simulink library "Controllers"  (R2013a)
settings: Solver=ode45  StartTime=0.0  StopTime=10.0  RelTol=1e-3
settings Model: Creator=Felipe  LastModifiedBy=Felipe

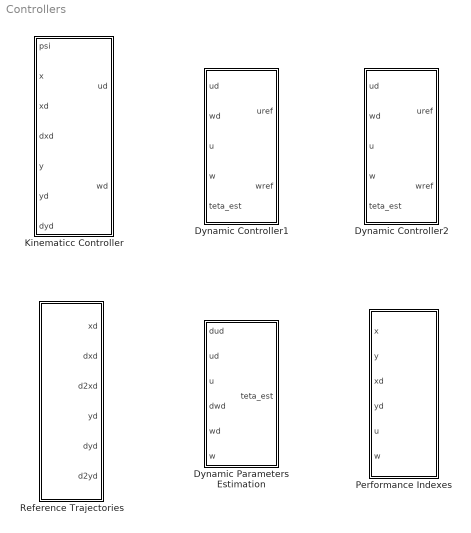
== system Controllers ==
  Dynamic Parameters Estimation : Subsystem  mask(Dynamic Parameters Estimation){ku=4, kw=4, lu=1, lw=1, inicia_adapt=50, theta=[0.30822 0.16922 -0.00058 0.80630 -0.00244 1.13994], gamma=[1.7 1.1 0.5 0.5 0.5 0.5], sig_mod=[0.0005 0.001 0.001 0.00006 0.001 0.000]}
      mask prompts: ku "Dynamic controller linear velocity gain: ku"; kw "Dynamic controller angular velocity gain: kw"; lu "Dynamic controller linear velocity saturation constant: lu"; lw "Dynamic controller angular velocity saturation constant: lw"; inicia_adapt "Time to begin parameter update: t[s]"; theta "Initial parameter estimates (1x6):"; gamma "Adaptation gains for parameter estimation (1x6):"; sig_mod "Sigma modification gains for parameter estimation (1x6):"
      mask help: This block implements a dynamic parameters estimatior to be used with the velocity-based dynamic compensation controller for differential-drive mobile robots.
      mask Help:
      | This block implements a dynamic parameters estimatior to be used with the velocity-based dynamic compensation controller for differential-drive mobile robots.
      | It receives the robot actual [u, w] and desired [ud, wd] values for linear and angular velocities, and the desired robot acceleration [dud, dwd]. Based on the velocity error, it adjusts the values of the estimated dynamic parameters [teta_est].
      | 
      | <b>Parameters:</b>
      | 
      | ku > 0 and kw > 0 are the dynamic controller gains.
      | lu > 0 and lw > 0 are the dynamic controller saturation constants.
      | t [s] (1x1): time to begin parameter update (before this time parameter estimates are kept constant)
      | gamma (1x6): adaptation gains for parameter estimation
      | Initial parameter estimates (1x6): Initial estimates for the dynamic parameters
      | 
      | <b>Inputs:</b>
      | 
      | dud (1x1): desired linear acceleration [m/s^2];
      | dwd (1x1): desired angular acceleration [rad/s^2];
      | ud (1x1): desired linear velocity [m/s] generated by the kinematic controller;
      | wd (1x1): desired angular velocity [rad/s] generated by the kinematic controller;
      | u (1x1): actual robot linear velocity [m/s];
      | w (1x1): actual robot angular velocity [rad/s];
      | 
      | 
      | <b>Outputs:</b>
      | 
      | teta_est (1x6): Estimated dynamic parameters for the mobile robot acoording to [1-3]:
      | [\theta_1 [s], \theta_2 [s], \theta_3 [sm/rad2], \theta_4, \theta_5 [s/m], \theta_6]
      | 
      | <b>Use:</b>
      | 
      | The inputs must recieve the reference signals for linear and angular velocities generated by a kinematic controller, and the actual robot linear and angular velocities.
      | The output [teta_est] is to be conected to a dynamic compensator controller.
      | 
      | <b>Notes:</b>
      | 
      | The following sets of parameters were obtained via identification for some differential-drive mobile robots:
      | 
      | [0.2604 0.2509 -0.000499 0.9965 0.00263 1.0768]; % Pioneer 3 with Sick LASER sensor
      | [0.5338 0.2168 -0.0134 0.9560 -0.0843 1.0590]; % Pioneer 3 without LASER sensor
      | [0.1992 0.13736 0.001954 0.9907 0.01554 0.9866]; % Pioneer 2 without onboard computer (no LASER sensor)
      | [0.3037 0.2768 -0.0004018 0.9835 0.003818 1.0725]; % Pioneer 2 with onboard computer (no LASER sensor)
      | [0.3759 0.0188 0.0128 1.0027 -0.0015 0.9808]; % Robotic wheelchair carring a 55kg person
      | [0.4263 0.0289 0.0058 0.9883 0.0134 0.9931]; % Robotic wheelchair carring a 125kg person
      | 
      | 
      | ------
      | For detailed information on the system, please refer to the following papers and thesis:
      | 
      | [1] MARTINS, F. N., Celeste, W. C., Carelli, R., Sarcinelli-Filho, M. and
      | Bastos-Filho, T. F. An Adaptive Dynamic Controller for Autonomous Mobile Robot
      | Trajectory Tracking. Control Engineering Practice, v. 16, p. 1354–1363, 2008.
      | doi: 10.1016/j.conengprac.2008.03.004
      | 
      | [2] MARTINS, F. N., Carelli, R., Sarcinelli-Filho, M. and Bastos-Filho, T. F.
      | Dynamic Modeling and Adaptive Dynamic Compensation for Unicycle-Like
      | Mobile Robots. 14th International Conference on Advanced Robotics -
      | ICAR 2009, Germany, June, 22-26, 2009.
      | 
      | [3] Thesis: "Modelagem e Compensacao da Dinamica de Robos Moveis e sua
      | Aplicacao em Controle de Formacao". Felipe Nascimento Martins. Tese de
      | Doutorado em Engenharia Eletrica - Automacao. UFES, 2009.
      | 
      | ---
      | Based on a prior work by Felipe Nascimento Martins and Wanderley Cardoso Celeste
      | UFES - Federal University of Espirito Santo, BRAZIL
      | 2006--2008
      | 
      | Author: Felipe Nascimento Martins
      | Federal Institute of Education, Science and Technology of Espirito Santo - IFES
      | NERA - Núcleo de Estudos em Robótica e Automação
      | http://nera.sr.ifes.edu.br
      | MAY/2013
      | Blog sobre robótica: www.nossosrobos.blogspot.com
  Dynamic Controller1 : Subsystem  mask(Dynamic Controller 1){ku=4, kw=4}
      mask prompts: ku "Linear velocity gain: ku"; kw "Angular velocity gain: kw"
      mask help: This block implements a velocity-based dynamic compensation controller for differential-drive mobile robots.
      mask Help:
      | This block implements a velocity-based dynamic compensation controller for differential-drive mobile robots.
      | It receives the references for linear and angular velocities [ud, wd] from the kinematic controller and generates another pair of linear and angular velocity commands [uref, wref] for the robot servos.
      | 
      | <b>Parameters:</b>
      | 
      | ku > 0 and kw > 0 are the controller gains.
      | 
      | <b>Inputs:</b>
      | 
      | ud (1x1): desired linear velocity [m/s] generated by the kinematic controller;
      | wd (1x1): desired angular velocity [rad/s] generated by the kinematic controller;
      | u (1x1): actual robot linear velocity [m/s];
      | w (1x1): actual robot angular velocity [rad/s];
      | teta_est (1x6): Estimated dynamic parameters for an specific mobile robot acoording to [1-3]:
      | [\theta_1 [s], \theta_2 [s], \theta_3 [sm/rad2], \theta_4, \theta_5 [s/m], \theta_6]
      | 
      | 
      | <b>Outputs:</b>
      | 
      | uref (1x1): reference for linear velocity [m/s]
      | wref (1x1): reference for angular velocity [rad/s]
      | 
      | <b>Use:</b>
      | 
      | The inputs must recieve the reference signals for linear and angular velocities generated by a kinematic controller, and the actual robot linear and angular velocities.
      | In order to perform correct dynamic compensation, the (1x6) vector of estimated dynamic parameters must be provided. This vector can be constant or can vary according to an adaptation rule.
      | 
      | The outputs [vref, wref] are to be conected to the robot.
      | 
      | 
      | <b>Notes:</b>
      | 
      | The following sets of parameters were obtained via identification for some differential-drive mobile robots:
      | 
      | [0.2604 0.2509 -0.000499 0.9965 0.00263 1.0768]; % Pioneer 3 with Sick LASER sensor
      | [0.5338 0.2168 -0.0134 0.9560 -0.0843 1.0590]; % Pioneer 3 without LASER sensor
      | [0.1992 0.13736 0.001954 0.9907 0.01554 0.9866]; % Pioneer 2 without onboard computer (no LASER sensor)
      | [0.3037 0.2768 -0.0004018 0.9835 0.003818 1.0725]; % Pioneer 2 with onboard computer (no LASER sensor)
      | [0.3759 0.0188 0.0128 1.0027 -0.0015 0.9808]; % Robotic wheelchair carring a 55kg person
      | [0.4263 0.0289 0.0058 0.9883 0.0134 0.9931]; % Robotic wheelchair carring a 125kg person
      | 
      | 
      | ------
      | For detailed information on the system, please refer to the following papers and thesis:
      | 
      | [1] MARTINS, F. N., Celeste, W. C., Carelli, R., Sarcinelli-Filho, M. and
      | Bastos-Filho, T. F. An Adaptive Dynamic Controller for Autonomous Mobile Robot
      | Trajectory Tracking. Control Engineering Practice, v. 16, p. 1354–1363, 2008.
      | doi: 10.1016/j.conengprac.2008.03.004
      | 
      | [2] MARTINS, F. N., Carelli, R., Sarcinelli-Filho, M. and Bastos-Filho, T. F.
      | Dynamic Modeling and Adaptive Dynamic Compensation for Unicycle-Like
      | Mobile Robots. 14th International Conference on Advanced Robotics -
      | ICAR 2009, Germany, June, 22-26, 2009.
      | 
      | [3] Thesis: "Modelagem e Compensacao da Dinamica de Robos Moveis e sua
      | Aplicacao em Controle de Formacao". Felipe Nascimento Martins. Tese de
      | Doutorado em Engenharia Eletrica - Automacao. UFES, 2009.
      | 
      | ---
      | Based on a prior work by Felipe Nascimento Martins and Wanderley Cardoso Celeste
      | UFES - Federal University of Espirito Santo, BRAZIL
      | 2006--2008
      | 
      | Author: Felipe Nascimento Martins
      | Federal Institute of Education, Science and Technology of Espirito Santo - IFES
      | NERA - Núcleo de Estudos em Robótica e Automação
      | http://nera.sr.ifes.edu.br
      | MAY/2013
      | Blog sobre robótica: www.nossosrobos.blogspot.com
  Dynamic Controller2 : Subsystem  mask(Dynamic Controller 2){ku=4, kw=4, lu=1, lw=1}
      mask prompts: ku "Linear velocity gain: ku"; kw "Angular velocity gain: kw"; lu "Linear velocity saturation constant: lu"; lw "Angular velocity saturation constant: lw"
      mask help: This block implements a velocity-based dynamic compensation controller for differential-drive mobile robots.
      mask Help:
      | This block implements a velocity-based dynamic compensation controller for differential-drive mobile robots.
      | It receives the references for linear and angular velocities [ud, wd] from the kinematic controller and generates another pair of linear and angular velocity commands [uref, wref] for the robot servos.
      | 
      | <b>Parameters:</b>
      | 
      | ku > 0 and kw > 0 are the controller gains.
      | lu > 0 and lw > 0 are saturation constants.
      | 
      | <b>Inputs:</b>
      | 
      | ud (1x1): desired linear velocity [m/s] generated by the kinematic controller;
      | wd (1x1): desired angular velocity [rad/s] generated by the kinematic controller;
      | u (1x1): actual robot linear velocity [m/s];
      | w (1x1): actual robot angular velocity [rad/s];
      | teta_est (1x6): Estimated dynamic parameters for an specific mobile robot acoording to [1-3]:
      | [\theta_1 [s], \theta_2 [s], \theta_3 [sm/rad2], \theta_4, \theta_5 [s/m], \theta_6]
      | 
      | 
      | <b>Outputs:</b>
      | 
      | uref (1x1): reference for linear velocity [m/s]
      | wref (1x1): reference for angular velocity [rad/s]
      | 
      | <b>Use:</b>
      | 
      | The inputs must recieve the reference signals for linear and angular velocities generated by a kinematic controller, and the actual robot linear and angular velocities.
      | In order to perform correct dynamic compensation, the (1x6) vector of estimated dynamic parameters must be provided. This vector can be constant or can vary according to an adaptation rule.
      | 
      | The outputs [vref, wref] are to be conected to the robot.
      | 
      | 
      | <b>Notes:</b>
      | 
      | The following sets of parameters were obtained via identification for some differential-drive mobile robots:
      | 
      | [0.2604 0.2509 -0.000499 0.9965 0.00263 1.0768]; % Pioneer 3 with Sick LASER sensor
      | [0.5338 0.2168 -0.0134 0.9560 -0.0843 1.0590]; % Pioneer 3 without LASER sensor
      | [0.1992 0.13736 0.001954 0.9907 0.01554 0.9866]; % Pioneer 2 without onboard computer (no LASER sensor)
      | [0.3037 0.2768 -0.0004018 0.9835 0.003818 1.0725]; % Pioneer 2 with onboard computer (no LASER sensor)
      | [0.3759 0.0188 0.0128 1.0027 -0.0015 0.9808]; % Robotic wheelchair carring a 55kg person
      | [0.4263 0.0289 0.0058 0.9883 0.0134 0.9931]; % Robotic wheelchair carring a 125kg person
      | 
      | 
      | ------
      | For detailed information on the system, please refer to the following papers and thesis:
      | 
      | [1] MARTINS, F. N., Celeste, W. C., Carelli, R., Sarcinelli-Filho, M. and
      | Bastos-Filho, T. F. An Adaptive Dynamic Controller for Autonomous Mobile Robot
      | Trajectory Tracking. Control Engineering Practice, v. 16, p. 1354–1363, 2008.
      | doi: 10.1016/j.conengprac.2008.03.004
      | 
      | [2] MARTINS, F. N., Carelli, R., Sarcinelli-Filho, M. and Bastos-Filho, T. F.
      | Dynamic Modeling and Adaptive Dynamic Compensation for Unicycle-Like
      | Mobile Robots. 14th International Conference on Advanced Robotics -
      | ICAR 2009, Germany, June, 22-26, 2009.
      | 
      | [3] Thesis: "Modelagem e Compensacao da Dinamica de Robos Moveis e sua
      | Aplicacao em Controle de Formacao". Felipe Nascimento Martins. Tese de
      | Doutorado em Engenharia Eletrica - Automacao. UFES, 2009.
      | 
      | ---
      | Based on a prior work by Felipe Nascimento Martins and Wanderley Cardoso Celeste
      | UFES - Federal University of Espirito Santo, BRAZIL
      | 2006--2008
      | 
      | Author: Felipe Nascimento Martins
      | Federal Institute of Education, Science and Technology of Espirito Santo - IFES
      | NERA - Núcleo de Estudos em Robótica e Automação
      | http://nera.sr.ifes.edu.br
      | MAY/2013
      | Blog sobre robótica: www.nossosrobos.blogspot.com
  Kinematicc Controller : Subsystem  mask(Kinematic Controller){kx=4, ky=4, lx=4, ly=4, a=0.2}
      mask prompts: kx "Controller gain: kx"; ky "Controller gain: ky"; lx "Saturation constant: lx"; ly "Saturation constant: ly"; a "Distance from the the point of interest to the center of the line that connects the traction wheels [m]"
      mask help: This block implements a controller for differential-drive mobile robots to follow a desired trajectory or to go to a goal point.
      mask Help:
      | This block implements a controller for differential-drive mobile robots to follow a desired trajectory or to go to a goal point.
      | 
      | The trajectory tracking controller is based on the inverse kinematics of the differential-drive robot, whereas only the position [x, y] of the point of interest is considered.
      | It generates references for linear and angular velocities [ud, wd] based on the robot's actual pose [x, y, psi] deseired position [xd, yd] and desired speed [dxd, dyd].
      | 
      | The constant "a" represents the distance of the point of interest [x, y] to the center of the line that connects the traction wheels.
      | 
      | <b>Parameters:</b>
      | 
      | kx > 0 and ky > 0: controller gains;
      | lx > 0 and ly > 0: saturation constants.
      | 
      | 
      | <b>Inputs:</b>
      | 
      | psi: actual robot orientation [rad] (psi=0 means the robot orientation is the same as the x axis);
      | x: actual robot position [m] in x axis;
      | xd: desired robot position [m] in x axis;
      | dxd: desired robot speed [m/s] in x axis;
      | y: actual robot position [m] in y axis;
      | yd: desired robot position [m] in y axis;
      | dyd: desired robot speed [m/s] in y axis;
      | 
      | <b>Outputs:</b>
      | 
      | ud: reference for linear velocity [m/s]
      | wd: reference for angular velocity [rad/s]
      | 
      | 
      | <b>Notes:</b>
      | 
      | If the deseired position [xd, yd] is constant and the desired speed [dxd, dyd] is zero, the controller works as a position controller: it drives the robot to a goal position [xd, yd].
      | 
      | ------
      | For detailed information on the system, please refer to the following papers and thesis:
      | 
      | [1] MARTINS, F. N., Celeste, W. C., Carelli, R., Sarcinelli-Filho, M. and
      | Bastos-Filho, T. F. An Adaptive Dynamic Controller for Autonomous Mobile Robot
      | Trajectory Tracking. Control Engineering Practice, v. 16, p. 1354–1363, 2008.
      | doi: 10.1016/j.conengprac.2008.03.004
      | 
      | [2] MARTINS, F. N., Carelli, R., Sarcinelli-Filho, M. and Bastos-Filho, T. F.
      | Dynamic Modeling and Adaptive Dynamic Compensation for Unicycle-Like
      | Mobile Robots. 14th International Conference on Advanced Robotics -
      | ICAR 2009, Germany, June, 22-26, 2009.
      | 
      | [3] Thesis: "Modelagem e Compensacao da Dinamica de Robos Moveis e sua
      | Aplicacao em Controle de Formacao". Felipe Nascimento Martins. Tese de
      | Doutorado em Engenharia Eletrica - Automacao. UFES, 2009.
      | 
      | ---
      | Based on a prior work by Felipe Nascimento Martins and Wanderley Cardoso Celeste
      | UFES - Federal University of Espirito Santo, BRAZIL
      | 2006--2008
      | 
      | Author: Felipe Nascimento Martins
      | Federal Institute of Education, Science and Technology of Espirito Santo - IFES
      | NERA - Núcleo de Estudos em Robótica e Automação
      | http://nera.sr.ifes.edu.br
      | MAY/2013
      | Blog sobre robótica: www.nossosrobos.blogspot.com
  Performance Indexes : Subsystem  mask(Performance Indexes){}
      mask help:
      | Calcultes the following performance indexes: IAE, ITAE, ISE, ITSE. Also calculates an Energy-based index.
      | Results are transfered to workspace variables: iae, itae, ise, itse, energy.
      mask Help:
      | Calcultes the following performance indexes: IAE, ITAE, ISE, ITSE. Also calculates an Energy-based index.
      | This block is intended to be used with mobile robot model and controllers in order to provide information to compare the performance of different controllers and gain sets.
      | 
      | Inputs:
      | x: actual robot position in x
      | y: actual robot position in y
      | xd: desired robot position in x
      | yd: desired robot position in y
      | u: actual robot linear velocity
      | w: actual robot angular velocity
      | 
      | Outputs:
      | Results are transfered to workspace variables: iae, itae, ise, itse, energy.
  Reference Trajectories : Subsystem  mask(Reference Trajectories){trajectory_type=2, wf=0.10, raio_ref_1=1, delta_raio=-0.1, t_delta_raio=60, xd=[2, 3]}
      mask prompts: trajectory_type "Trajectory type: 1=Circle, 2=Eight, 3=Line, 4=Fixed Point"; wf "Angular speed for circle and eight [rad/s]"; raio_ref_1 "Radius for circle and eight (each side) [m]"; delta_raio "Radius variation (circle only)"; t_delta_raio "Time between radius variation (circle only) [s]"; xd "Goal position (for fixed point only) (1x2)"
      mask help: Generates reference values of position, velocity and acceleration.
      mask Help:
      | Generates reference values of position, velocity and acceleration.
      | This block is intended to be used with mobile robot trajectory tracking kinematic controller.
      | 
      | Available references:
      | - Circular trajectory with 2 different radius;
      | - Eight-shape trajectory;
      | - Linear trajectory;
      | - Fixed point.
      | 
      | 
      | <b> Parameters:</b>
      | 
      | Trajectory type: 1=Circle, 2=Eight, 3=Line, 4=Fixed Point
      | Angular speed for circle and eight (1x1) [rad/s]
      | Radius for circle and eight (each side) (1x1)[m]
      | Radius variation (circle only) delta_raio (1x1) [m]
      | Time between radius variation (circle only) (1x1) [s]
      | 
      | <b> Outputs: </b>
      | 
      | xd: desired robot position [m] in x axis;
      | dxd: desired robot speed [m/s] in x axis;
      | d2xd: desired robot acceleration [m/s^2] in x axis;
      | yd: desired robot position [m] in y axis;
      | dyd: desired robot speed [m/s] in y axis;
      | d2yd: desired robot acceleration [m/s^2] in y axis;

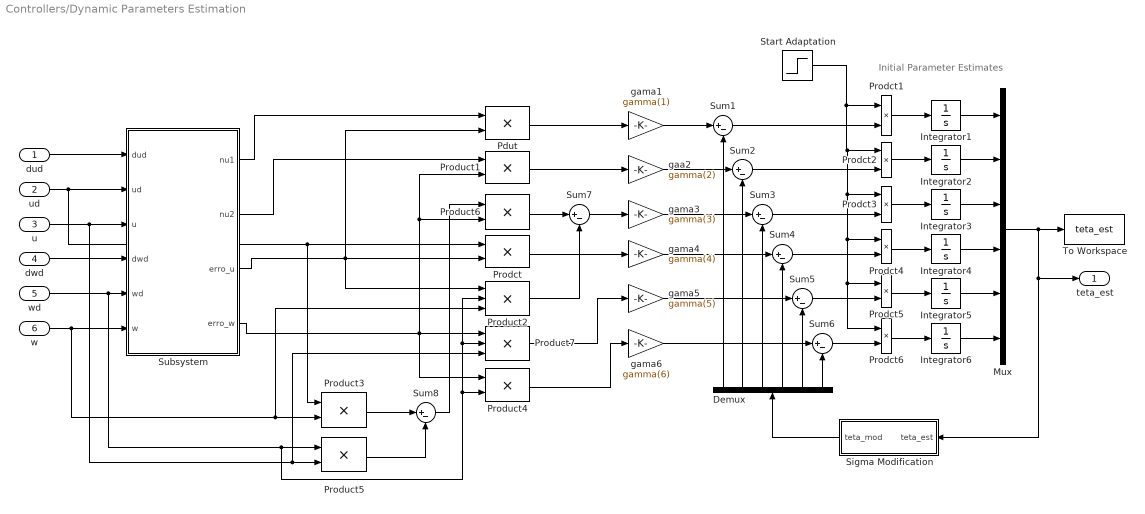
== system Controllers/Dynamic Parameters Estimation ==
  note: Initial Parameter
      | Estimates
  dud : Inport
  ud : Inport  Port=2
  u : Inport  Port=3
  dwd : Inport  Port=4
  wd : Inport  Port=5
  w : Inport  Port=6
  Demux : Demux  Outputs=6
  Integrator1 : Integrator  InitialCondition=theta(1)
  Integrator2 : Integrator  InitialCondition=theta(2)
  Integrator3 : Integrator  InitialCondition=theta(3)
  Integrator4 : Integrator  InitialCondition=theta(4)
  Integrator5 : Integrator  InitialCondition=theta(5)
  Integrator6 : Integrator  InitialCondition=theta(6)
  Mux : Mux  Inputs=6
  Pdut : Product  SaturateOnIntegerOverflow=on  OutDataTypeStr=Inherit: Same as first input
  Prodct{,1..6} (7 alike) : Product  SaturateOnIntegerOverflow=on  OutDataTypeStr=Inherit: Same as first input
  Product{1,3..6} (5 alike) : Product  SaturateOnIntegerOverflow=on  OutDataTypeStr=Inherit: Same as first input
  Product2 : Product  Inputs=3  SaturateOnIntegerOverflow=on  OutDataTypeStr=Inherit: Same as first input
  Product7 : Product  Inputs=3  SaturateOnIntegerOverflow=on  OutDataTypeStr=Inherit: Same as first input
  Sigma Modification : Subsystem
  Start Adaptation : Step  Time=inicia_adapt  SampleTime=0
  Subsystem : Subsystem
  Sum{1..8} (8 alike) : Sum  Inputs=|+-  SaturateOnIntegerOverflow=on
  To Workspace : ToWorkspace  VariableName=teta_est  SampleTime=-1
  gaa2 : Gain  Gain=gamma(2)  SaturateOnIntegerOverflow=on  OutDataTypeStr=Inherit: Same as input  ParamDataTypeStr=Inherit: Same as input
  gama1 : Gain  Gain=gamma(1)  SaturateOnIntegerOverflow=on  OutDataTypeStr=Inherit: Same as input  ParamDataTypeStr=Inherit: Same as input
  gama3 : Gain  Gain=gamma(3)  SaturateOnIntegerOverflow=on  OutDataTypeStr=Inherit: Same as input  ParamDataTypeStr=Inherit: Same as input
  gama4 : Gain  Gain=gamma(4)  SaturateOnIntegerOverflow=on  OutDataTypeStr=Inherit: Same as input  ParamDataTypeStr=Inherit: Same as input
  gama5 : Gain  Gain=gamma(5)  SaturateOnIntegerOverflow=on  OutDataTypeStr=Inherit: Same as input  ParamDataTypeStr=Inherit: Same as input
  gama6 : Gain  Gain=gamma(6)  SaturateOnIntegerOverflow=on  OutDataTypeStr=Inherit: Same as input  ParamDataTypeStr=Inherit: Same as input
  teta_est : Outport
  wires:
  dud/1 -> Subsystem/1(dud)
  dwd/1 -> Subsystem/4(dwd)
  Subsystem/1(nu1) -> Pdut/1
  Subsystem/2(nu2) -> Product1/1
  Pdut/1 -> gama1/1
  Product1/1 -> gaa2/1
  Prodct/1 -> gama4/1
  Product4/1 -> gama6/1
  Integrator1/1 -> Mux/1
  Integrator2/1 -> Mux/2
  Integrator3/1 -> Mux/3
  Integrator4/1 -> Mux/4
  Integrator5/1 -> Mux/5
  Integrator6/1 -> Mux/6
  Mux/1 -> To Workspace/1, teta_est/1, Sigma Modification/1(teta_est)
  Prodct1/1 -> Integrator1/1
  Prodct2/1 -> Integrator2/1
  Prodct3/1 -> Integrator3/1
  Prodct4/1 -> Integrator4/1
  Prodct5/1 -> Integrator5/1
  Prodct6/1 -> Integrator6/1
  Sigma Modification/1(teta_mod) -> Demux/1
  Sum1/1 -> Prodct1/2
  gama1/1 -> Sum1/1
  Demux/1 -> Sum1/2
  gaa2/1 -> Sum2/1
  Sum2/1 -> Prodct2/2
  Demux/2 -> Sum2/2
  Sum3/1 -> Prodct3/2
  gama3/1 -> Sum3/1
  Demux/3 -> Sum3/2
  gama4/1 -> Sum4/1
  Sum4/1 -> Prodct4/2
  Demux/4 -> Sum4/2
  Sum5/1 -> Prodct5/2
  gama5/1 -> Sum5/1
  Demux/5 -> Sum5/2
  gama6/1 -> Sum6/1
  Demux/6 -> Sum6/2
  Sum6/1 -> Prodct6/2
  Sum7/1 -> gama3/1
  Product2/1 -> Sum7/2
  Product3/1 -> Sum8/1
  Product5/1 -> Sum8/2
  Sum8/1 -> Product6/1
  Product6/1 -> Sum7/1
  Product7/1 -> gama5/1
  Start Adaptation/1 -> Prodct4/1, Prodct5/1, Prodct6/1, Prodct3/1, Prodct2/1, Prodct1/1
  ud/1 -> Subsystem/2(ud), Product3/1, Prodct/1
  u/1 -> Product7/3, Product5/2, Subsystem/3(u)
  wd/1 -> Product4/2, Product7/2, Product2/2, Product5/1, Subsystem/5(wd)
  w/1 -> Product2/3, Product3/2, Subsystem/6(w)
  Subsystem/3(erro_u) -> Product2/1, Pdut/2, Prodct/2
  Subsystem/4(erro_w) -> Product1/2, Product6/2, Product4/1, Product7/1

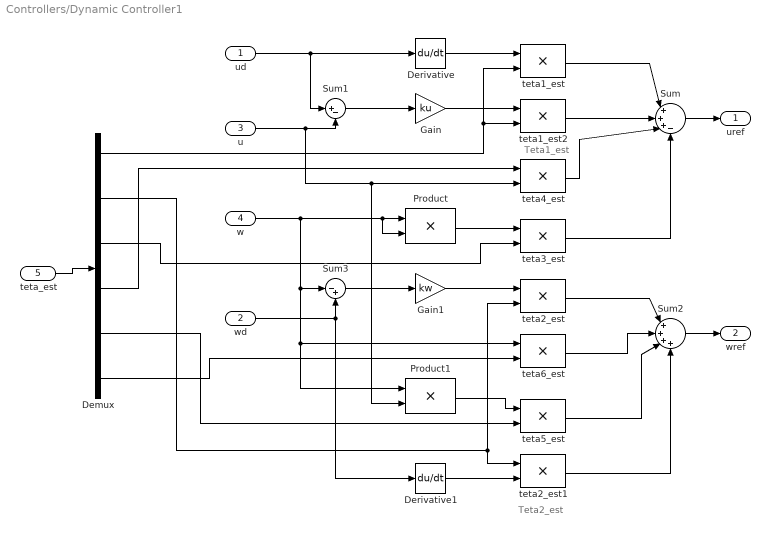
== system Controllers/Dynamic Controller1 ==
  note: Teta2_est
  note: Teta1_est
  ud : Inport
  wd : Inport  Port=2
  u : Inport  Port=3
  w : Inport  Port=4
  teta_est : Inport  Port=5
  Demux : Demux  Outputs=6
  Derivative : Derivative
  Derivative1 : Derivative
  Gain : Gain  Gain=ku  SaturateOnIntegerOverflow=on  OutDataTypeStr=Inherit: Same as input  ParamDataTypeStr=Inherit: Same as input
  Gain1 : Gain  Gain=kw  SaturateOnIntegerOverflow=on  OutDataTypeStr=Inherit: Same as input  ParamDataTypeStr=Inherit: Same as input
  Product : Product  SaturateOnIntegerOverflow=on  OutDataTypeStr=Inherit: Same as first input
  Product1 : Product  SaturateOnIntegerOverflow=on  OutDataTypeStr=Inherit: Same as first input
  Sum : Sum  Inputs=|+++-  SaturateOnIntegerOverflow=on
  Sum1 : Sum  Inputs=|+-  SaturateOnIntegerOverflow=on
  Sum2 : Sum  Inputs=|++++  SaturateOnIntegerOverflow=on
  Sum3 : Sum  Inputs=|-+  SaturateOnIntegerOverflow=on
  teta1_est : Product  SaturateOnIntegerOverflow=on  OutDataTypeStr=Inherit: Same as first input
  teta1_est2 : Product  SaturateOnIntegerOverflow=on  OutDataTypeStr=Inherit: Same as first input
  teta2_est : Product  SaturateOnIntegerOverflow=on  OutDataTypeStr=Inherit: Same as first input
  teta2_est1 : Product  SaturateOnIntegerOverflow=on  OutDataTypeStr=Inherit: Same as first input
  teta3_est : Product  SaturateOnIntegerOverflow=on  OutDataTypeStr=Inherit: Same as first input
  teta4_est : Product  SaturateOnIntegerOverflow=on  OutDataTypeStr=Inherit: Same as first input
  teta5_est : Product  SaturateOnIntegerOverflow=on  OutDataTypeStr=Inherit: Same as first input
  teta6_est : Product  SaturateOnIntegerOverflow=on  OutDataTypeStr=Inherit: Same as first input
  uref : Outport
  wref : Outport  Port=2
  wires:
  Sum/1 -> uref/1
  Sum2/1 -> wref/1
  Sum1/1 -> Gain/1
  teta1_est/1 -> Sum/1
  Product/1 -> teta3_est/1
  teta3_est/1 -> Sum/4
  Sum3/1 -> Gain1/1
  teta6_est/1 -> Sum2/2
  Product1/1 -> teta5_est/1
  teta1_est2/1 -> Sum/2
  teta_est/1 -> Demux/1
  teta4_est/1 -> Sum/3
  Demux/3 -> teta3_est/2
  teta2_est/1 -> Sum2/1
  Demux/6 -> teta6_est/2
  teta5_est/1 -> Sum2/3
  Demux/5 -> teta5_est/2
  teta2_est1/1 -> Sum2/4
  Derivative/1 -> teta1_est/1
  Derivative1/1 -> teta2_est1/2
  Gain/1 -> teta1_est2/1
  Gain1/1 -> teta2_est/1
  Demux/1 -> teta1_est/2, teta1_est2/2
  ud/1 -> Sum1/1, Derivative/1
  u/1 -> Sum1/2, teta4_est/2, Product1/2
  w/1 -> teta6_est/1, Product1/1, Sum3/1, Product/2, Product/1
  wd/1 -> Derivative1/1, Sum3/2
  Demux/2 -> teta2_est/2, teta2_est1/1
  Demux/4 -> teta4_est/1

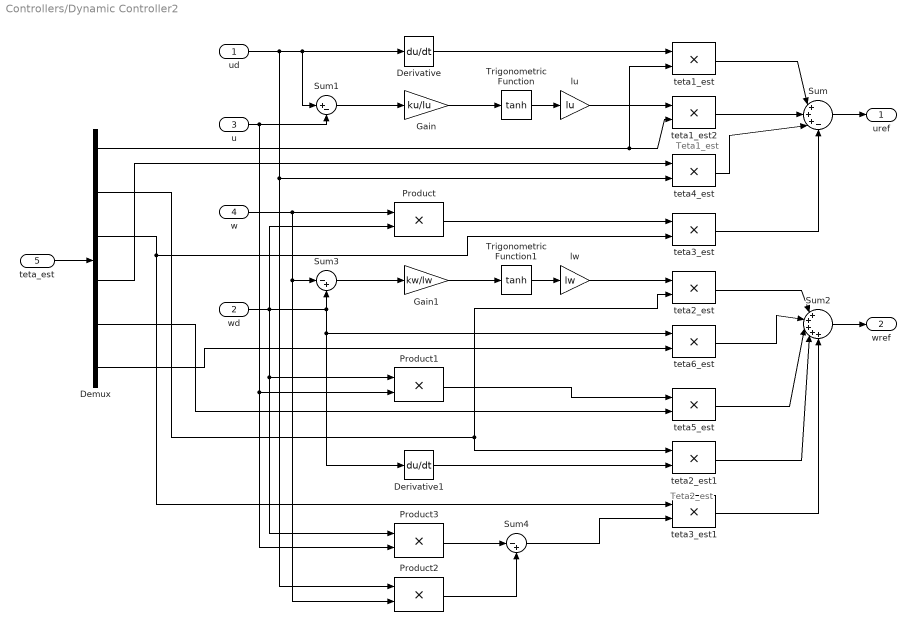
== system Controllers/Dynamic Controller2 ==
  note: Teta2_est
  note: Teta1_est
  ud : Inport
  wd : Inport  Port=2
  u : Inport  Port=3
  w : Inport  Port=4
  teta_est : Inport  Port=5
  Demux : Demux  Outputs=6
  Derivative : Derivative
  Derivative1 : Derivative
  Gain : Gain  Gain=ku/lu  SaturateOnIntegerOverflow=on  OutDataTypeStr=Inherit: Same as input  ParamDataTypeStr=Inherit: Same as input
  Gain1 : Gain  Gain=kw/lw  SaturateOnIntegerOverflow=on  OutDataTypeStr=Inherit: Same as input  ParamDataTypeStr=Inherit: Same as input
  Product{,1..3} (4 alike) : Product  SaturateOnIntegerOverflow=on  OutDataTypeStr=Inherit: Same as first input
  Sum : Sum  Inputs=|+++-  SaturateOnIntegerOverflow=on
  Sum1 : Sum  Inputs=|+-  SaturateOnIntegerOverflow=on
  Sum2 : Sum  Inputs=|+++++  SaturateOnIntegerOverflow=on
  Sum3 : Sum  Inputs=|-+  SaturateOnIntegerOverflow=on
  Sum4 : Sum  Inputs=|-+  SaturateOnIntegerOverflow=on
  Trigonometric Function : Trigonometry  Operator=tanh
  Trigonometric Function1 : Trigonometry  Operator=tanh
  lu : Gain  Gain=lu  SaturateOnIntegerOverflow=on  OutDataTypeStr=Inherit: Same as input  ParamDataTypeStr=Inherit: Same as input
  lw : Gain  Gain=lw  SaturateOnIntegerOverflow=on  OutDataTypeStr=Inherit: Same as input  ParamDataTypeStr=Inherit: Same as input
  teta1_est : Product  SaturateOnIntegerOverflow=on  OutDataTypeStr=Inherit: Same as first input
  teta1_est2 : Product  SaturateOnIntegerOverflow=on  OutDataTypeStr=Inherit: Same as first input
  teta2_est : Product  SaturateOnIntegerOverflow=on  OutDataTypeStr=Inherit: Same as first input
  teta2_est1 : Product  SaturateOnIntegerOverflow=on  OutDataTypeStr=Inherit: Same as first input
  teta3_est : Product  SaturateOnIntegerOverflow=on  OutDataTypeStr=Inherit: Same as first input
  teta3_est1 : Product  SaturateOnIntegerOverflow=on  OutDataTypeStr=Inherit: Same as first input
  teta4_est : Product  SaturateOnIntegerOverflow=on  OutDataTypeStr=Inherit: Same as first input
  teta5_est : Product  SaturateOnIntegerOverflow=on  OutDataTypeStr=Inherit: Same as first input
  teta6_est : Product  SaturateOnIntegerOverflow=on  OutDataTypeStr=Inherit: Same as first input
  uref : Outport
  wref : Outport  Port=2
  wires:
  Sum/1 -> uref/1
  Sum2/1 -> wref/1
  Sum1/1 -> Gain/1
  teta1_est/1 -> Sum/1
  Product/1 -> teta3_est/1
  teta3_est/1 -> Sum/4
  Sum3/1 -> Gain1/1
  teta6_est/1 -> Sum2/2
  Product1/1 -> teta5_est/1
  teta1_est2/1 -> Sum/2
  teta_est/1 -> Demux/1
  teta4_est/1 -> Sum/3
  Demux/3 -> teta3_est1/1, teta3_est/2
  teta2_est/1 -> Sum2/1
  Demux/6 -> teta6_est/2
  teta5_est/1 -> Sum2/3
  Demux/5 -> teta5_est/2
  teta2_est1/1 -> Sum2/4
  Derivative/1 -> teta1_est/1
  Derivative1/1 -> teta2_est1/2
  Demux/1 -> teta1_est/2, teta1_est2/2
  ud/1 -> Product2/1, teta4_est/2, Sum1/1, Derivative/1
  u/1 -> Sum1/2, Product3/2, Product1/2
  w/1 -> Product2/2, Sum3/1, Product/1
  wd/1 -> Product3/1, Product1/1, Product/2, teta6_est/1, Derivative1/1, Sum3/2
  Demux/2 -> teta2_est/2, teta2_est1/1
  Demux/4 -> teta4_est/1
  Trigonometric Function/1 -> lu/1
  lu/1 -> teta1_est2/1
  Gain/1 -> Trigonometric Function/1
  Trigonometric Function1/1 -> lw/1
  lw/1 -> teta2_est/1
  Gain1/1 -> Trigonometric Function1/1
  teta3_est1/1 -> Sum2/5
  Sum4/1 -> teta3_est1/2
  Product3/1 -> Sum4/1
  Product2/1 -> Sum4/2

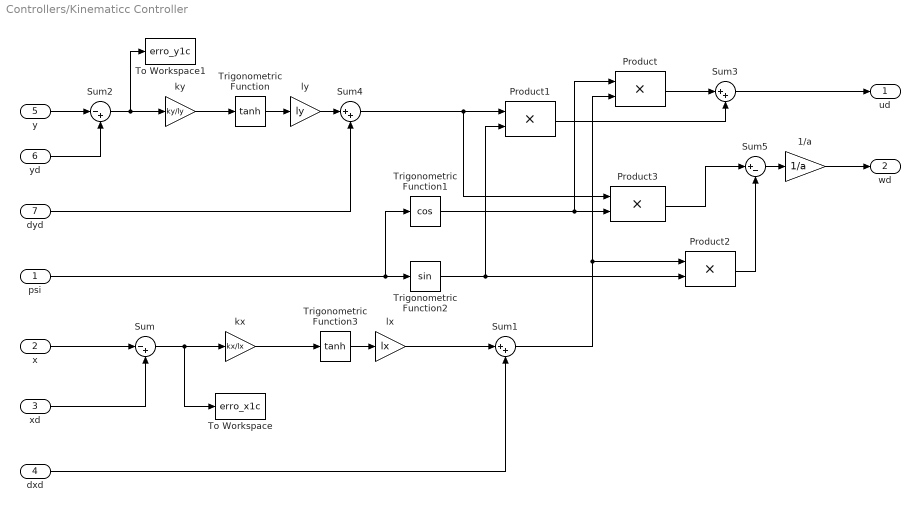
== system Controllers/Kinematicc Controller ==
  psi : Inport
  x : Inport  Port=2
  xd : Inport  Port=3
  dxd : Inport  Port=4
  y : Inport  Port=5
  yd : Inport  Port=6
  dyd : Inport  Port=7
  1/a : Gain  Gain=1/a  SaturateOnIntegerOverflow=on  OutDataTypeStr=Inherit: Same as input  ParamDataTypeStr=Inherit: Same as input
  Product{,1..3} (4 alike) : Product  SaturateOnIntegerOverflow=on  OutDataTypeStr=Inherit: Same as first input
  Sum : Sum  Inputs=|-+  SaturateOnIntegerOverflow=on
  Sum1 : Sum  Inputs=|++  SaturateOnIntegerOverflow=on
  Sum2 : Sum  Inputs=|-+  SaturateOnIntegerOverflow=on
  Sum3 : Sum  Inputs=|++  SaturateOnIntegerOverflow=on
  Sum4 : Sum  Inputs=|++  SaturateOnIntegerOverflow=on
  Sum5 : Sum  Inputs=|+-  SaturateOnIntegerOverflow=on
  To Workspace : ToWorkspace  VariableName=erro_x1c  SampleTime=-1
  To Workspace1 : ToWorkspace  VariableName=erro_y1c  SampleTime=-1
  Trigonometric Function : Trigonometry  Operator=tanh
  Trigonometric Function1 : Trigonometry  Operator=cos
  Trigonometric Function2 : Trigonometry
  Trigonometric Function3 : Trigonometry  Operator=tanh
  kx : Gain  Gain=kx/lx  SaturateOnIntegerOverflow=on  OutDataTypeStr=Inherit: Same as input  ParamDataTypeStr=Inherit: Same as input
  ky : Gain  Gain=ky/ly  SaturateOnIntegerOverflow=on  OutDataTypeStr=Inherit: Same as input  ParamDataTypeStr=Inherit: Same as input
  lx : Gain  Gain=lx  SaturateOnIntegerOverflow=on  OutDataTypeStr=Inherit: Same as input  ParamDataTypeStr=Inherit: Same as input
  ly : Gain  Gain=ly  SaturateOnIntegerOverflow=on  OutDataTypeStr=Inherit: Same as input  ParamDataTypeStr=Inherit: Same as input
  ud : Outport
  wd : Outport  Port=2
  wires:
  Sum5/1 -> 1/a/1
  Product2/1 -> Sum5/2
  Product3/1 -> Sum5/1
  Product1/1 -> Sum3/2
  Product/1 -> Sum3/1
  Sum2/1 -> To Workspace1/1, ky/1
  Sum1/1 -> Product/2, Product2/1
  psi/1 -> Trigonometric Function1/1, Trigonometric Function2/1
  x/1 -> Sum/1
  xd/1 -> Sum/2
  yd/1 -> Sum2/2
  Trigonometric Function3/1 -> lx/1
  lx/1 -> Sum1/1
  Trigonometric Function/1 -> ly/1
  ly/1 -> Sum4/1
  dyd/1 -> Sum4/2
  dxd/1 -> Sum1/2
  Sum3/1 -> ud/1
  1/a/1 -> wd/1
  Trigonometric Function2/1 -> Product1/2, Product2/2
  Sum4/1 -> Product3/1, Product1/1
  y/1 -> Sum2/1
  Sum/1 -> To Workspace/1, kx/1
  Trigonometric Function1/1 -> Product/1, Product3/2
  ky/1 -> Trigonometric Function/1
  kx/1 -> Trigonometric Function3/1

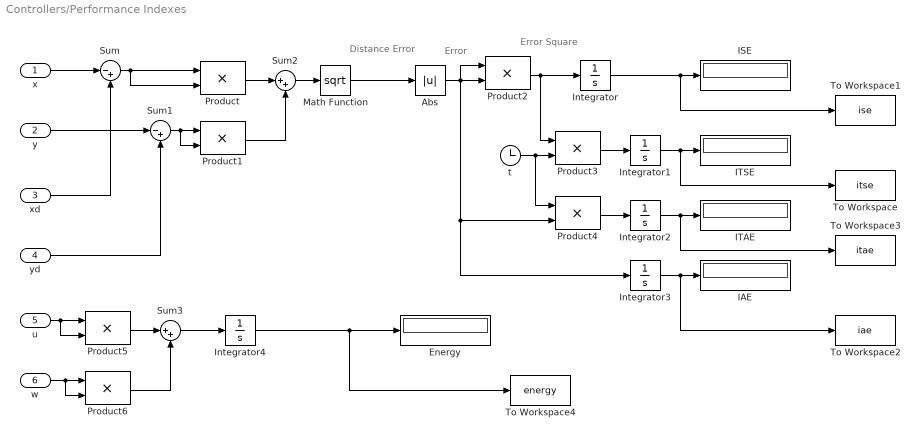
== system Controllers/Performance Indexes ==
  note: Error
      | Square
  note: Error
  note: Distance
      | Error
  x : Inport
  y : Inport  Port=2
  xd : Inport  Port=3
  yd : Inport  Port=4
  u : Inport  Port=5
  w : Inport  Port=6
  Abs : Abs  SaturateOnIntegerOverflow=on
  Energy : Display
  IAE : Display
  ISE : Display
  ITAE : Display
  ITSE : Display
  Integrator{,1..4} (5 alike) : Integrator
  Math Function : Math  Operator=sqrt  SaturateOnIntegerOverflow=on
  Product{,1..6} (7 alike) : Product  SaturateOnIntegerOverflow=on  OutDataTypeStr=Inherit: Same as first input
  Sum : Sum  Inputs=|-+  SaturateOnIntegerOverflow=on
  Sum1 : Sum  Inputs=|-+  SaturateOnIntegerOverflow=on
  Sum2 : Sum  Inputs=|++  SaturateOnIntegerOverflow=on
  Sum3 : Sum  Inputs=|++  SaturateOnIntegerOverflow=on
  To Workspace : ToWorkspace  VariableName=itse  SampleTime=-1
  To Workspace1 : ToWorkspace  VariableName=ise  SampleTime=-1
  To Workspace2 : ToWorkspace  VariableName=iae  SampleTime=-1
  To Workspace3 : ToWorkspace  VariableName=itae  SampleTime=-1
  To Workspace4 : ToWorkspace  VariableName=energy  SampleTime=-1
  t : Clock
  wires:
  Integrator4/1 -> To Workspace4/1, Energy/1
  w/1 -> Product6/2, Product6/1
  u/1 -> Product5/2, Product5/1
  Sum3/1 -> Integrator4/1
  Product6/1 -> Sum3/2
  Product5/1 -> Sum3/1
  Abs/1 -> Integrator3/1, Product4/2, Product2/1, Product2/2
  Integrator3/1 -> To Workspace2/1, IAE/1
  Product4/1 -> Integrator2/1
  Integrator2/1 -> To Workspace3/1, ITAE/1
  Product3/1 -> Integrator1/1
  Integrator1/1 -> To Workspace/1, ITSE/1
  t/1 -> Product4/1, Product3/2
  Integrator/1 -> To Workspace1/1, ISE/1
  Product2/1 -> Product3/1, Integrator/1
  Math Function/1 -> Abs/1
  Sum2/1 -> Math Function/1
  Product1/1 -> Sum2/2
  Product/1 -> Sum2/1
  Sum1/1 -> Product1/2, Product1/1
  Sum/1 -> Product/2, Product/1
  yd/1 -> Sum1/2
  y/1 -> Sum1/1
  xd/1 -> Sum/2
  x/1 -> Sum/1

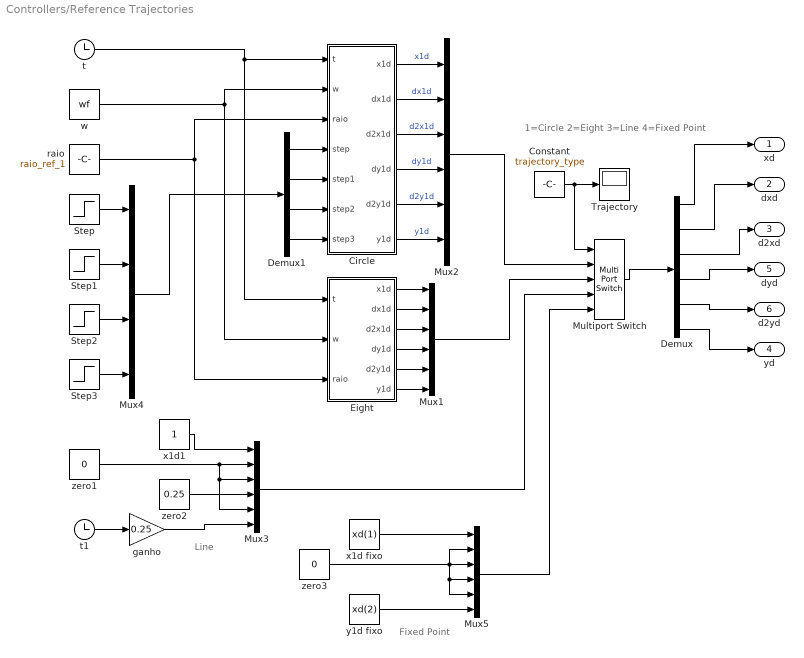
== system Controllers/Reference Trajectories ==
  note: Fixed Point
  note: Line
  note: 1=Circle
      | 2=Eight
      | 3=Line
      | 4=Fixed Point
  Circle : Subsystem
  Constant : Constant  Value=trajectory_type
  Demux : Demux  Outputs=6
  Demux1 : Demux
  Eight : Subsystem
  Multiport Switch : MultiPortSwitch  Inputs=4  SaturateOnIntegerOverflow=on
  Mux{1..3,5} (4 alike) : Mux  Inputs=6
  Mux4 : Mux
  Step : Step  Time=t_delta_raio  After=delta_raio  SampleTime=0
  Step1 : Step  Time=t_delta_raio*2  After=-delta_raio  SampleTime=0
  Step2 : Step  Time=t_delta_raio*3  After=delta_raio  SampleTime=0
  Step3 : Step  Time=t_delta_raio*4  After=-delta_raio  SampleTime=0
  Trajectory : Display
      settings: Format=decimal (Stored Integer)
  ganho : Gain  Gain=0.25  SaturateOnIntegerOverflow=on  OutDataTypeStr=Inherit: Same as input  ParamDataTypeStr=Inherit: Same as input
  raio : Constant  Value=raio_ref_1
  t : Clock
  t1 : Clock
  w : Constant  Value=wf
  x1d fixo : Constant  Value=xd(1)
  x1d1 : Constant
  y1d fixo : Constant  Value=xd(2)
  zero1 : Constant  Value=0
  zero2 : Constant  Value=0.25
  zero3 : Constant  Value=0
  xd : Outport
  dxd : Outport  Port=2
  d2xd : Outport  Port=3
  yd : Outport  Port=4
  dyd : Outport  Port=5
  d2yd : Outport  Port=6
  wires:
  zero3/1 -> Mux5/5, Mux5/4, Mux5/2, Mux5/3
  x1d fixo/1 -> Mux5/1
  y1d fixo/1 -> Mux5/6
  Mux5/1 -> Multiport Switch/5
  Mux3/1 -> Multiport Switch/4
  Multiport Switch/1 -> Demux/1
  Mux4/1 -> Demux1/1
  Demux1/4 -> Circle/7(step3)
  Demux1/3 -> Circle/6(step2)
  Demux1/2 -> Circle/5(step1)
  Demux1/1 -> Circle/4(step)
  Step3/1 -> Mux4/4
  Step2/1 -> Mux4/3
  Step1/1 -> Mux4/2
  Step/1 -> Mux4/1
  zero2/1 -> Mux3/4
  ganho/1 -> Mux3/6
  zero1/1 -> Mux3/5, Mux3/3, Mux3/2
  t1/1 -> ganho/1
  x1d1/1 -> Mux3/1
  Eight/6(y1d) -> Mux1/6
  Eight/5(d2y1d) -> Mux1/5
  Eight/4(dy1d) -> Mux1/4
  Eight/3(d2x1d) -> Mux1/3
  Eight/2(dx1d) -> Mux1/2
  Eight/1(x1d) -> Mux1/1
  Circle/6(y1d) -> Mux2/6  "y1d"
  Circle/5(d2y1d) -> Mux2/5  "d2y1d"
  Circle/4(dy1d) -> Mux2/4  "dy1d"
  Circle/3(d2x1d) -> Mux2/3  "d2x1d"
  Circle/2(dx1d) -> Mux2/2  "dx1d"
  Circle/1(x1d) -> Mux2/1  "x1d"
  Demux/6 -> yd/1
  Demux/5 -> d2yd/1
  Demux/4 -> dyd/1
  Demux/3 -> d2xd/1
  Demux/2 -> dxd/1
  Demux/1 -> xd/1
  Constant/1 -> Trajectory/1, Multiport Switch/1
  Mux2/1 -> Multiport Switch/2
  Mux1/1 -> Multiport Switch/3
  w/1 -> Eight/2(w), Circle/2(w)
  raio/1 -> Eight/3(raio), Circle/3(raio)
  t/1 -> Eight/1(t), Circle/1(t)

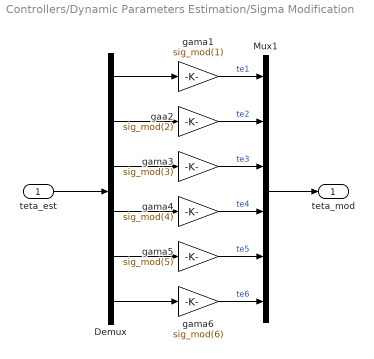
== system Controllers/Dynamic Parameters Estimation/Sigma Modification ==
  teta_est : Inport
  Demux : Demux  Outputs=6
  Mux1 : Mux  Inputs=6
  gaa2 : Gain  Gain=sig_mod(2)  SaturateOnIntegerOverflow=on  OutDataTypeStr=Inherit: Same as input  ParamDataTypeStr=Inherit: Same as input
  gama1 : Gain  Gain=sig_mod(1)  SaturateOnIntegerOverflow=on  OutDataTypeStr=Inherit: Same as input  ParamDataTypeStr=Inherit: Same as input
  gama3 : Gain  Gain=sig_mod(3)  SaturateOnIntegerOverflow=on  OutDataTypeStr=Inherit: Same as input  ParamDataTypeStr=Inherit: Same as input
  gama4 : Gain  Gain=sig_mod(4)  SaturateOnIntegerOverflow=on  OutDataTypeStr=Inherit: Same as input  ParamDataTypeStr=Inherit: Same as input
  gama5 : Gain  Gain=sig_mod(5)  SaturateOnIntegerOverflow=on  OutDataTypeStr=Inherit: Same as input  ParamDataTypeStr=Inherit: Same as input
  gama6 : Gain  Gain=sig_mod(6)  SaturateOnIntegerOverflow=on  OutDataTypeStr=Inherit: Same as input  ParamDataTypeStr=Inherit: Same as input
  teta_mod : Outport
  wires:
  teta_est/1 -> Demux/1
  Demux/1 -> gama1/1
  Demux/2 -> gaa2/1
  Demux/3 -> gama3/1
  Demux/4 -> gama4/1
  Demux/5 -> gama5/1
  Demux/6 -> gama6/1
  gama1/1 -> Mux1/1  "te1"
  gaa2/1 -> Mux1/2  "te2"
  gama3/1 -> Mux1/3  "te3"
  gama4/1 -> Mux1/4  "te4"
  gama5/1 -> Mux1/5  "te5"
  gama6/1 -> Mux1/6  "te6"
  Mux1/1 -> teta_mod/1

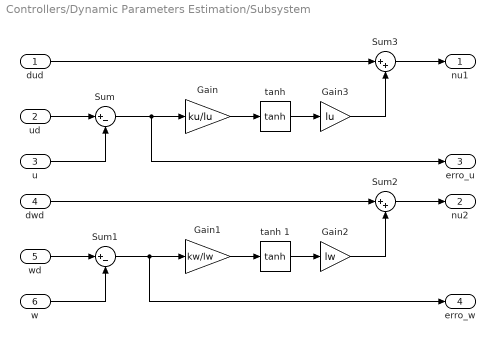
== system Controllers/Dynamic Parameters Estimation/Subsystem ==
  dud : Inport
  ud : Inport  Port=2
  u : Inport  Port=3
  dwd : Inport  Port=4
  wd : Inport  Port=5
  w : Inport  Port=6
  Gain : Gain  Gain=ku/lu  SaturateOnIntegerOverflow=on  OutDataTypeStr=Inherit: Same as input  ParamDataTypeStr=Inherit: Same as input
  Gain1 : Gain  Gain=kw/lw  SaturateOnIntegerOverflow=on  OutDataTypeStr=Inherit: Same as input  ParamDataTypeStr=Inherit: Same as input
  Gain2 : Gain  Gain=lw  SaturateOnIntegerOverflow=on  OutDataTypeStr=Inherit: Same as input  ParamDataTypeStr=Inherit: Same as input
  Gain3 : Gain  Gain=lu  SaturateOnIntegerOverflow=on  OutDataTypeStr=Inherit: Same as input  ParamDataTypeStr=Inherit: Same as input
  Sum : Sum  Inputs=|+-  SaturateOnIntegerOverflow=on
  Sum1 : Sum  Inputs=|+-  SaturateOnIntegerOverflow=on
  Sum2 : Sum  Inputs=|++  SaturateOnIntegerOverflow=on
  Sum3 : Sum  Inputs=|++  SaturateOnIntegerOverflow=on
  "tanh " : Trigonometry  Operator=tanh
  tanh 1 : Trigonometry  Operator=tanh
  nu1 : Outport
  nu2 : Outport  Port=2
  erro_u : Outport  Port=3
  erro_w : Outport  Port=4
  wires:
  wd/1 -> Sum1/1
  w/1 -> Sum1/2
  Sum1/1 -> Gain1/1, erro_w/1
  dwd/1 -> Sum2/1
  Sum3/1 -> nu1/1
  Gain/1 -> "tanh "/1
  "tanh "/1 -> Gain3/1
  ud/1 -> Sum/1
  u/1 -> Sum/2
  Sum/1 -> Gain/1, erro_u/1
  Gain3/1 -> Sum3/2
  Gain1/1 -> tanh 1/1
  tanh 1/1 -> Gain2/1
  Gain2/1 -> Sum2/2
  Sum2/1 -> nu2/1
  dud/1 -> Sum3/1

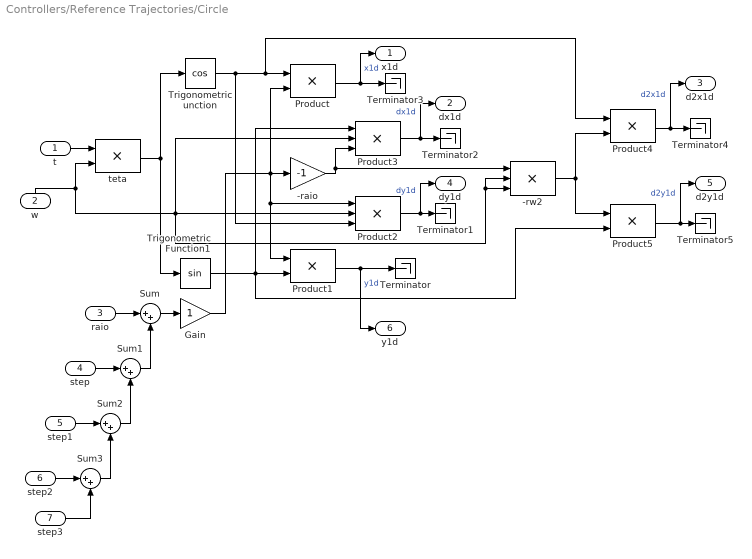
== system Controllers/Reference Trajectories/Circle ==
  t : Inport
  w : Inport  Port=2
  raio : Inport  Port=3
  step : Inport  Port=4
  step1 : Inport  Port=5
  step2 : Inport  Port=6
  step3 : Inport  Port=7
  -raio : Gain  Gain=-1  SaturateOnIntegerOverflow=on  OutDataTypeStr=Inherit: Same as input  ParamDataTypeStr=Inherit: Same as input
  -rw2 : Product  Inputs=3  SaturateOnIntegerOverflow=on  OutDataTypeStr=Inherit: Same as first input
  Gain : Gain  SaturateOnIntegerOverflow=on  OutDataTypeStr=Inherit: Same as input  ParamDataTypeStr=Inherit: Same as input
  Product{,1,4..5} (4 alike) : Product  SaturateOnIntegerOverflow=on  OutDataTypeStr=Inherit: Same as first input
  Product2 : Product  Inputs=3  SaturateOnIntegerOverflow=on  OutDataTypeStr=Inherit: Same as first input
  Product3 : Product  Inputs=3  SaturateOnIntegerOverflow=on  OutDataTypeStr=Inherit: Same as first input
  Sum{,1..3} (4 alike) : Sum  Inputs=|++  SaturateOnIntegerOverflow=on
  Terminator{,1..5} (6 alike) : Terminator
  Trigonometric Function1 : Trigonometry
  Trigonometric unction : Trigonometry  Operator=cos
  teta : Product  SaturateOnIntegerOverflow=on  OutDataTypeStr=Inherit: Same as first input
  x1d : Outport
  dx1d : Outport  Port=2
  d2x1d : Outport  Port=3
  dy1d : Outport  Port=4
  d2y1d : Outport  Port=5
  y1d : Outport  Port=6
  wires:
  step3/1 -> Sum3/2
  step2/1 -> Sum3/1
  step1/1 -> Sum2/1
  step/1 -> Sum1/1
  raio/1 -> Sum/1
  t/1 -> teta/1
  Sum3/1 -> Sum2/2
  Sum2/1 -> Sum1/2
  Sum1/1 -> Sum/2
  Sum/1 -> Gain/1
  Gain/1 -> Product/2, Product2/1, Product1/1, -raio/1
  Product5/1 -> d2y1d/1, Terminator5/1  "d2y1d"
  Product4/1 -> d2x1d/1, Terminator4/1  "d2x1d"
  -rw2/1 -> Product5/1, Product4/2
  -raio/1 -> -rw2/1, Product3/3
  Product3/1 -> dx1d/1, Terminator2/1  "dx1d"
  Product2/1 -> dy1d/1, Terminator1/1  "dy1d"
  teta/1 -> Trigonometric Function1/1, Trigonometric unction/1
  Product1/1 -> Terminator/1, y1d/1  "y1d"
  Product/1 -> Terminator3/1, x1d/1  "x1d"
  w/1 -> teta/2, Product3/2, -rw2/3, -rw2/2, Product2/2
  Trigonometric Function1/1 -> Product5/2, Product3/1, Product1/2
  Trigonometric unction/1 -> Product/1, Product4/1, Product2/3

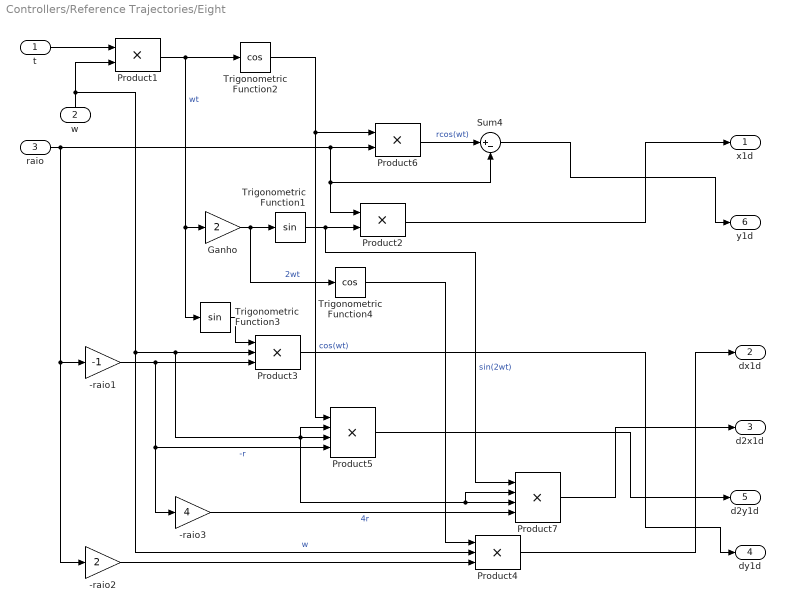
== system Controllers/Reference Trajectories/Eight ==
  t : Inport
  w : Inport  Port=2
  raio : Inport  Port=3
  -raio1 : Gain  Gain=-1  SaturateOnIntegerOverflow=on  OutDataTypeStr=Inherit: Same as input  ParamDataTypeStr=Inherit: Same as input
  -raio2 : Gain  Gain=2  SaturateOnIntegerOverflow=on  OutDataTypeStr=Inherit: Same as input  ParamDataTypeStr=Inherit: Same as input
  -raio3 : Gain  Gain=4  SaturateOnIntegerOverflow=on  OutDataTypeStr=Inherit: Same as input  ParamDataTypeStr=Inherit: Same as input
  Ganho : Gain  Gain=2  SaturateOnIntegerOverflow=on  OutDataTypeStr=Inherit: Same as input  ParamDataTypeStr=Inherit: Same as input
  Product1 : Product  SaturateOnIntegerOverflow=on  OutDataTypeStr=Inherit: Same as first input
  Product2 : Product  SaturateOnIntegerOverflow=on  OutDataTypeStr=Inherit: Same as first input
  Product3 : Product  Inputs=3  SaturateOnIntegerOverflow=on  OutDataTypeStr=Inherit: Same as first input
  Product4 : Product  Inputs=3  SaturateOnIntegerOverflow=on  OutDataTypeStr=Inherit: Same as first input
  Product5 : Product  Inputs=4  SaturateOnIntegerOverflow=on  OutDataTypeStr=Inherit: Same as first input
  Product6 : Product  SaturateOnIntegerOverflow=on  OutDataTypeStr=Inherit: Same as first input
  Product7 : Product  Inputs=4  SaturateOnIntegerOverflow=on  OutDataTypeStr=Inherit: Same as first input
  Sum4 : Sum  Inputs=|+-  SaturateOnIntegerOverflow=on
  Trigonometric Function1 : Trigonometry
  Trigonometric Function2 : Trigonometry  Operator=cos
  Trigonometric Function3 : Trigonometry
  Trigonometric Function4 : Trigonometry  Operator=cos
  x1d : Outport
  dx1d : Outport  Port=2
  d2x1d : Outport  Port=3
  dy1d : Outport  Port=4
  d2y1d : Outport  Port=5
  y1d : Outport  Port=6
  wires:
  Product5/1 -> d2y1d/1
  Product7/1 -> d2x1d/1
  Product3/1 -> dy1d/1
  Product4/1 -> dx1d/1
  Sum4/1 -> y1d/1
  Product2/1 -> x1d/1
  -raio3/1 -> Product7/4  "4r"
  Trigonometric Function4/1 -> Product4/1
  -raio2/1 -> Product4/3
  -raio1/1 -> -raio3/1, Product5/4, Product3/3  "-r"
  Trigonometric Function3/1 -> Product3/1
  Trigonometric Function1/1 -> Product7/1, Product2/2  "sin(2wt)"
  Ganho/1 -> Trigonometric Function4/1, Trigonometric Function1/1  "2wt"
  Product6/1 -> Sum4/1  "rcos(wt)"
  Trigonometric Function2/1 -> Product5/1, Product6/1  "cos(wt)"
  raio/1 -> -raio2/1, -raio1/1, Product2/1, Sum4/2, Product6/2
  Product1/1 -> Trigonometric Function3/1, Ganho/1, Trigonometric Function2/1  "wt"
  w/1 -> Product7/2, Product7/3, Product5/2, Product5/3, Product3/2, Product4/2, Product1/2  "w"
  t/1 -> Product1/1
